simulink model "MultiLoop_mode1_old"  (R2021b)
settings: Solver=ode45  StartTime=0.0  StopTime=72  FixedStep=Ts_base  MinStep=1e-6  RelTol=1e-6
PreLoadFcn:
  | Mode_1_Init
InitFcn:
  | hApp = TEP_app;
  | %hApp = fault_selection_App;
StartFcn:
  | disp('simulator')
  | blk = 'MultiLoop_mode1/TE Plant/Pressure';
  | event = 'PostOutputs';
  | listener = @(app, event) updateGUI(hApp);
  | h = add_exec_event_listener(blk, event, listener);
StopFcn:
  | %TEplot
undefined symbols (not defined in the file or in its folder): r1_0, r4_0, Ts_base, Ts_save
libraries: TElib x17
settings Model: PacingRate=0.001000  Creator=ricker  LastModifiedBy=Omar
settings SolverCC: AlgebraicLoopSolver=TrustRegion
settings DataIOCC: LoadInitialState=on  SaveFinalState=on  SaveFormat=Structure  SignalLoggingSaveFormat=ModelDataLogs  SaveOutput=off  SignalLogging=off  SaveTime=off  ReturnWorkspaceOutputs=off  SignalLoggingName=sigsOut
settings OptimizationCC: InitFltsAndDblsToZero=on  LifeSpan=inf
settings DebuggingCC: SaveWithParameterizedLinksMsg=none  UnderspecifiedInitializationDetection=Classic  MergeDetectMultiDrivingBlocksExec=none  SignalResolutionControl=TryResolveAllWithWarning  MultiTaskDSMMsg=warning  MultiTaskCondExecSysMsg=none  FcnCallInpInsideContextMsg=warning  SFUnexpectedBacktrackingDiag=warning  SFNoUnconditionalDefaultTransitionDiag=warning  SFExecutionAtInitializationDiag=none  SFMachineParentedDataDiag=warning  ArithmeticOperatorsInVariantConditions=warning
settings HardwareCC: ProdBitPerPointer=32  ProdBitPerSizeT=32  ProdBitPerPtrDiffT=32  ProdLargestAtomicFloat=None  ProdIntDivRoundTo=Undefined  ProdEndianess=Unspecified  ProdWordSize=32  ProdHWDeviceType=32-bit Generic  TargetUnknown=on
settings ModelReferenceCC: PropagateSignalLabelsOutOfModel=off
settings SFSimCC: SimUseLocalCustomCode=off  CustomCodeUndefinedFunction=UseInterfaceOnly
settings RTWCC: RTWUseLocalCustomCode=off
settings CodeAppCC: StateflowObjectComments=on
settings GRTTargetCC: TargetFcnLib=ansi_tfl_tmw.mat  TargetLangStandard=C89/C90 (ANSI)  CombineOutputUpdateFcns=off  GRTInterface=on
settings ConfigComp: CovMetricSettings=dw  CovSaveCumulativeToWorkspaceVar=on  CovSaveSingleToWorkspaceVar=on  CovExternalEMLEnable=off  CovSFcnEnable=off

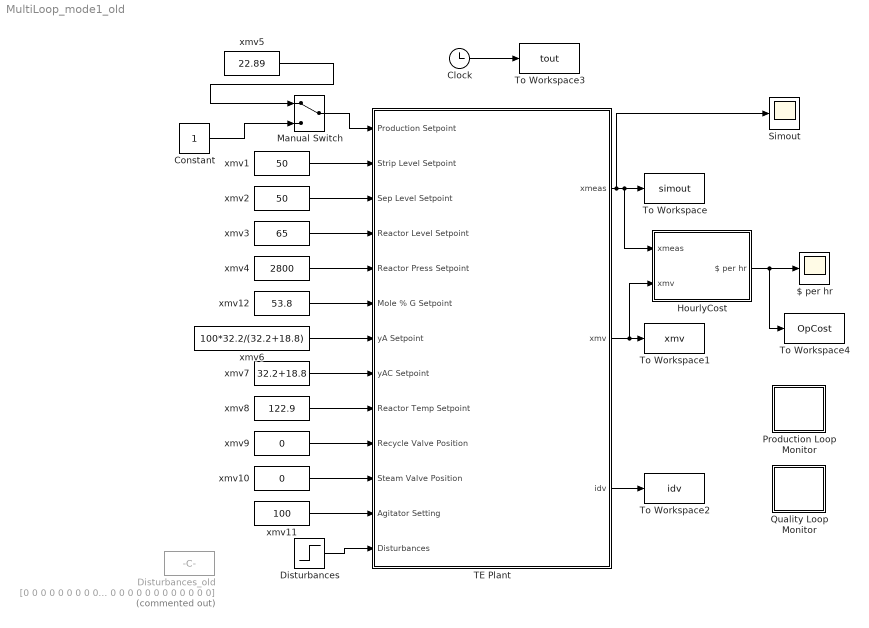
== system MultiLoop_mode1_old ==
  $ per hr : Scope
  Clock : Clock
  Constant : Constant
  Disturbances : Step  Time=0  Before=[0 0 0 0 0 0 0 0 0 0 0 0 0 0 0 0 0 0 0 0 0 0 0 0 0 0 0 0]  After=[0 0 0 0 0 0 0 0 0 0 0 0 0 0 0 0 0 0 0 0 0 0 0 0 0 0 0 0]  SampleTime=0
  Disturbances_old : Constant  Commented=on  Value=[0 0 0 0 0 0 0 0 0 0 0 0 0 0 0 0 0 0 0 0 0 0 0 0 0 0 0 0]
  HourlyCost : Subsystem
  Manual Switch : ManualSwitch
  Production Loop Monitor : Subsystem
  Quality Loop Monitor : Subsystem
  Simout : Scope
  TE Plant : Subsystem
  To Workspace : ToWorkspace  VariableName=simout  SampleTime=Ts_save
  To Workspace1 : ToWorkspace  VariableName=xmv  SampleTime=Ts_save
  To Workspace2 : ToWorkspace  VariableName=idv  SampleTime=Ts_save
  To Workspace3 : ToWorkspace  VariableName=tout  SampleTime=Ts_save
  To Workspace4 : ToWorkspace  VariableName=OpCost  SampleTime=Ts_save
  xmv1 : Constant  Value=50
  xmv10 : Constant  Value=0
  xmv11 : Constant  Value=100
  xmv12 : Constant  Value=53.8
  xmv2 : Constant  Value=50
  xmv3 : Constant  Value=65
  xmv4 : Constant  Value=2800
  xmv5 : Constant  Value=22.89
  xmv6 : Constant  Value=100*32.2/(32.2+18.8)
  xmv7 : Constant  Value=32.2+18.8
  xmv8 : Constant  Value=122.9
  xmv9 : Constant  Value=0
  wires:
  TE Plant/1(xmeas) -> Simout/1, To Workspace/1, HourlyCost/1(xmeas)
  xmv1/1 -> TE Plant/2(Strip Level Setpoint)
  xmv2/1 -> TE Plant/3(Sep Level Setpoint)
  xmv3/1 -> TE Plant/4(Reactor Level Setpoint)
  xmv4/1 -> TE Plant/5(Reactor Press Setpoint)
  xmv8/1 -> TE Plant/9(Reactor Temp Setpoint)
  xmv6/1 -> TE Plant/7(yA Setpoint)
  xmv7/1 -> TE Plant/8(yAC Setpoint)
  TE Plant/2(xmv) -> To Workspace1/1, HourlyCost/2(xmv)
  TE Plant/3(idv) -> To Workspace2/1
  Clock/1 -> To Workspace3/1
  HourlyCost/1($ per hr) -> $ per hr/1, To Workspace4/1
  xmv9/1 -> TE Plant/10(Recycle Valve Position)
  xmv10/1 -> TE Plant/11(Steam Valve Position)
  xmv11/1 -> TE Plant/12(Agitator Setting)
  xmv12/1 -> TE Plant/6(Mole % G Setpoint)
  xmv5/1 -> Manual Switch/1
  Disturbances/1 -> TE Plant/13(Disturbances)
  Constant/1 -> Manual Switch/2
  Manual Switch/1 -> TE Plant/1(Production Setpoint)

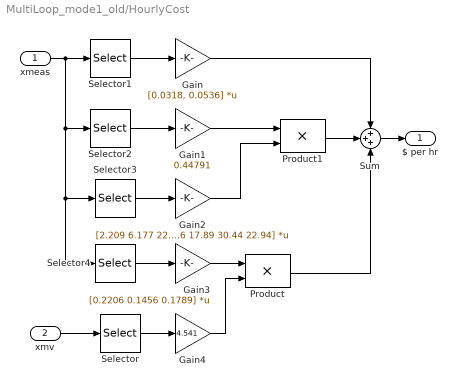
== system MultiLoop_mode1_old/HourlyCost ==
  xmeas : Inport  PortDimensions=41
  xmv : Inport  Port=2  PortDimensions=12
  Gain : Gain  Gain=[0.0318, 0.0536]  Multiplication=Matrix(K*u)  SaturateOnIntegerOverflow=on  OutDataTypeStr=Inherit: Same as input  ParamDataTypeStr=Inherit: Same as input
  Gain1 : Gain  Gain=0.44791  SaturateOnIntegerOverflow=on  OutDataTypeStr=Inherit: Same as input  ParamDataTypeStr=Inherit: Same as input
  Gain2 : Gain  Gain=[2.209 6.177 22.06 14.56 17.89 30.44 22.94]  Multiplication=Matrix(K*u)  SaturateOnIntegerOverflow=on  OutDataTypeStr=Inherit: Same as input  ParamDataTypeStr=Inherit: Same as input
  Gain3 : Gain  Gain=[0.2206 0.1456 0.1789]  Multiplication=Matrix(K*u)  SaturateOnIntegerOverflow=on  OutDataTypeStr=Inherit: Same as input  ParamDataTypeStr=Inherit: Same as input
  Gain4 : Gain  Gain=4.541  SaturateOnIntegerOverflow=on  OutDataTypeStr=Inherit: Same as input  ParamDataTypeStr=Inherit: Same as input
  Product : Product  SaturateOnIntegerOverflow=on  OutDataTypeStr=Inherit: Same as first input
  Product1 : Product  SaturateOnIntegerOverflow=on  OutDataTypeStr=Inherit: Same as first input
  Selector : Selector  InputPortWidth=12  IndexOptions=Index vector (dialog)  Indices=8  OutputSizes=1
  Selector1 : Selector  InputPortWidth=41  IndexOptions=Index vector (dialog)  Indices=[19 20]  OutputSizes=1
  Selector2 : Selector  InputPortWidth=41  IndexOptions=Index vector (dialog)  Indices=[10]  OutputSizes=1
  Selector3 : Selector  InputPortWidth=41  IndexOptions=Index vector (dialog)  Indices=[29, 31:36]  OutputSizes=1
  Selector4 : Selector  InputPortWidth=41  IndexOptions=Index vector (dialog)  Indices=[37:39]  OutputSizes=1
  Sum : Sum  Inputs=+++  SaturateOnIntegerOverflow=on
  $ per hr : Outport
  wires:
  xmv/1 -> Selector/1
  xmeas/1 -> Selector1/1, Selector2/1, Selector3/1, Selector4/1
  Selector1/1 -> Gain/1
  Selector2/1 -> Gain1/1
  Selector3/1 -> Gain2/1
  Selector4/1 -> Gain3/1
  Selector/1 -> Gain4/1
  Gain3/1 -> Product/1
  Gain4/1 -> Product/2
  Sum/1 -> $ per hr/1
  Product/1 -> Sum/3
  Gain/1 -> Sum/1
  Product1/1 -> Sum/2
  Gain1/1 -> Product1/1
  Gain2/1 -> Product1/2

== system MultiLoop_mode1_old/Production Loop Monitor ==
  Mux2 : Mux  Inputs=2
  Production : Scope
  wires:
  Mux2/1 -> Production/1
  [xmeas17] -> Mux2/2
  [Prodsp] -> Mux2/1

== system MultiLoop_mode1_old/Quality Loop Monitor ==
  Mux2 : Mux  Inputs=2
  Quality : Scope
  wires:
  [PctGsp] -> Mux2/1
  [xmeas40] -> Mux2/2
  Mux2/1 -> Quality/1

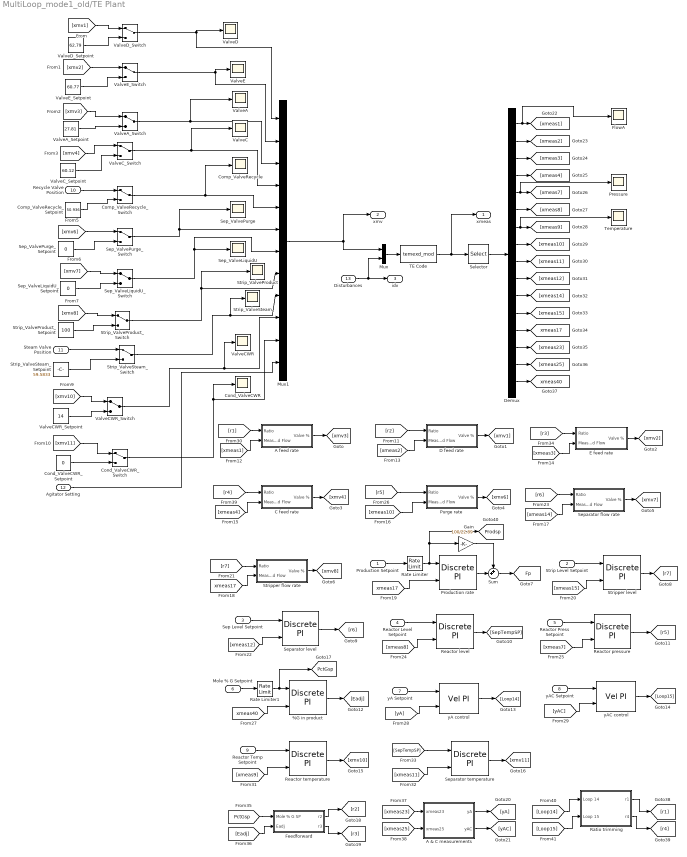
== system MultiLoop_mode1_old/TE Plant ==
  Production Setpoint : Inport
  Strip Level Setpoint : Inport  Port=2
  Sep Level Setpoint : Inport  Port=3
  Reactor Level Setpoint : Inport  Port=4
  Reactor Press Setpoint : Inport  Port=5
  Mole % G Setpoint : Inport  Port=6
  yA Setpoint : Inport  Port=7
  yAC Setpoint : Inport  Port=8
  Reactor Temp Setpoint : Inport  Port=9
  Recycle Valve Position : Inport  Port=10
  Steam Valve Position : Inport  Port=11
  Agitator Setting : Inport  Port=12
  Disturbances : Inport  Port=13
  %G in product : TElib/Discrete PI  Kc=-0.4  Ti=100/60  Ts=Ts_base  x0=Eadj_0  Hi=inf  Lo=-inf
  A & C measurements : Subsystem
  A feed rate : Subsystem
  C feed rate : Subsystem
  Comp_ValveRecycle : Scope
  Comp_ValveRecycle_Setpoint : Constant  Value=50.936
  Comp_ValveRecycle_Switch : ManualSwitch
  Cond_ValveCWR : Scope
  Cond_ValveCWR_Setpoint : Constant  Value=0
  Cond_ValveCWR_Switch : ManualSwitch
  D feed rate : Subsystem
  Demux : Demux  Outputs=16
      settings: DisplayOption=none
  E feed rate : Subsystem
  Feedforward : Subsystem
  FlowA : Scope
  Gain : Gain  Gain=100/22.89  SaturateOnIntegerOverflow=on  OutDataTypeStr=Inherit: Same as input  ParamDataTypeStr=Inherit: Same as input
  Mux : Mux  Inputs=2
  Mux1 : Mux  Inputs=12
  Pressure : Scope
  Production rate : TElib/Discrete PI  Kc=3.2  Ti=120/60  Ts=Ts_base  x0=0  Hi=30  Lo=-30
  Purge rate : Subsystem
  Rate Limiter : RateLimiter  RisingSlewLimit=0.3*22.95/24  FallingSlewLimit=-0.3*22.95/24
  Rate Limiter1 : RateLimiter  RisingSlewLimit=50/24  FallingSlewLimit=-50/24
  Ratio trimming : Subsystem
  Reactor level : TElib/Discrete PI  Kc=0.8  Ti=60/60  Ts=Ts_base  x0=SP17_0  Hi=120  Lo=0
  Reactor pressure : TElib/Discrete PI  Kc=-1e-4  Ti=20/60  Ts=Ts_base  x0=r5_0  Hi=100  Lo=0
  Reactor temperature : TElib/Discrete PI  Kc=-8  Ti=7.5/60  Ts=Ts_base  x0=xmv10_0  Hi=100  Lo=0
  Selector : Selector  InputPortWidth=41  IndexOptions=Index vector (dialog)  Indices=[1:4, 7:12, 14, 15, 17, 23, 25, 40]  OutputSizes=1
  Sep_ValveLiquidU : Scope
  Sep_ValveLiquidU_Setpoint : Constant  Value=0
  Sep_ValveLiquidU_Switch : ManualSwitch
  Sep_ValvePurge : Scope
  Sep_ValvePurge_Setpoint : Constant  Value=0
  Sep_ValvePurge_Switch : ManualSwitch
  Separator flow rate : Subsystem
  Separator level : TElib/Discrete PI  Kc=-1e-3  Ti=200/60  Ts=Ts_base  x0=r6_0  Hi=100  Lo=0
  Separator temperature : TElib/Discrete PI  Kc=-4  Ti=15/60  Ts=Ts_base  x0=xmv11_0  Hi=100  Lo=0
  Strip_ValveProduct : Scope
  Strip_ValveProduct_Setpoint : Constant  Value=100
  Strip_ValveProduct_Switch : ManualSwitch
  Strip_ValveSteam : Scope
  Strip_ValveSteam_Setpoint : Constant  Value=59.5833
  Strip_ValveSteam_Switch : ManualSwitch
  Stripper flow rate : Subsystem
  Stripper level : TElib/Discrete PI  Kc=-2e-4  Ti=200/60  Ts=Ts_base  x0=r7_0  Hi=100  Lo=0
  Sum : Sum  Inputs=++|  SaturateOnIntegerOverflow=on
  TE Code : S-Function  FunctionName=temexd_mod  SFunctionDeploymentMode=off  EnableBusSupport=off
  Temperature : Scope
  ValveA : Scope
  ValveA_Setpoint : Constant  Value=27.81
  ValveA_Switch : ManualSwitch
  ValveC : Scope
  ValveCWR : Scope
  ValveCWR_Setpoint : Constant  Value=14
  ValveCWR_Switch : ManualSwitch
  ValveC_Setpoint : Constant  Value=60.12
  ValveC_Switch : ManualSwitch
  ValveD : Scope
  ValveD_Setpoint : Constant  Value=62.79
  ValveD_Switch : ManualSwitch
  ValveE : Scope
  ValveE_Setpoint : Constant  Value=60.77
  ValveE_Switch : ManualSwitch
  yA control : TElib/Discrete PI/Vel PI  Kc=2e-4  Ti=1  Ts=0.1
  yAC control : TElib/Discrete PI/Vel PI  Kc=3e-4  Ti=2  Ts=0.1
  xmeas : Outport
  xmv : Outport  Port=2
  idv : Outport  Port=3
  tag scope: Fp=global, PctGsp=global, Prodsp=global, xmeas17=global, xmeas40=global
  wires:
  Mux/1 -> TE Code/1
  Disturbances/1 -> Mux/2, idv/1
  TE Code/1 -> xmeas/1, Selector/1
  [xmv1] -> ValveD_Switch/1
  Recycle Valve Position/1 -> Comp_ValveRecycle_Switch/1
  [xmv6] -> Sep_ValvePurge_Switch/1
  [xmv7] -> Sep_ValveLiquidU_Switch/1
  [xmv8] -> Strip_ValveProduct_Switch/1
  Steam Valve Position/1 -> Strip_ValveSteam_Switch/1
  [xmv10] -> ValveCWR_Switch/1
  [xmv11] -> Cond_ValveCWR_Switch/1
  Agitator Setting/1 -> Mux1/12
  A feed rate/1(Valve %) -> [xmv3]
  [xmeas1] -> A feed rate/2(Measured Flow)
  D feed rate/1(Valve %) -> [xmv1]
  [xmeas2] -> D feed rate/2(Measured Flow)
  E feed rate/1(Valve %) -> [xmv2]
  [xmeas3] -> E feed rate/2(Measured Flow)
  C feed rate/1(Valve %) -> [xmv4]
  [xmeas4] -> C feed rate/2(Measured Flow)
  Purge rate/1(Valve %) -> [xmv6]
  [xmeas10] -> Purge rate/2(Measured Flow)
  Separator flow rate/1(Valve %) -> [xmv7]
  [xmeas14] -> Separator flow rate/2(Measured Flow)
  Stripper flow rate/1(Valve %) -> [xmv8]
  [xmeas17] -> Stripper flow rate/2(Measured Flow)
  [xmeas17] -> Production rate/2
  [xmeas15] -> Stripper level/2
  Strip Level Setpoint/1 -> Stripper level/1
  Stripper level/1 -> [r7]
  [r7] -> Stripper flow rate/1(Ratio)
  [xmeas12] -> Separator level/2
  Sep Level Setpoint/1 -> Separator level/1
  Separator level/1 -> [r6]
  [r6] -> Separator flow rate/1(Ratio)
  [xmeas8] -> Reactor level/2
  Reactor Level Setpoint/1 -> Reactor level/1
  Reactor level/1 -> [SepTempSP]
  [xmeas7] -> Reactor pressure/2
  Reactor Press Setpoint/1 -> Reactor pressure/1
  Reactor pressure/1 -> [r5]
  [r5] -> Purge rate/1(Ratio)
  [xmeas40] -> %G in product/2
  %G in product/1 -> [Eadj]
  [yA] -> yA control/2
  yA Setpoint/1 -> yA control/1
  yA control/1 -> [Loop14]
  [yAC] -> yAC control/2
  yAC Setpoint/1 -> yAC control/1
  yAC control/1 -> [Loop15]
  [r1] -> A feed rate/1(Ratio)
  [xmeas9] -> Reactor temperature/2
  Reactor Temp Setpoint/1 -> Reactor temperature/1
  Reactor temperature/1 -> [xmv10]
  [xmeas11] -> Separator temperature/2
  [SepTempSP] -> Separator temperature/1
  Separator temperature/1 -> [xmv11]
  [r3] -> E feed rate/1(Ratio)
  [PctGsp] -> Feedforward/1(Mole % G SP)
  [Eadj] -> Feedforward/2(Eadj)
  Feedforward/1(r2) -> [r2]
  Feedforward/2(r3) -> [r3]
  [xmeas23] -> A & C measurements/1(xmeas23)
  [xmeas25] -> A & C measurements/2(xmeas25)
  A & C measurements/1(yA) -> [yA]
  A & C measurements/2(yAC) -> [yAC]
  Mux1/1 -> Mux/1, xmv/1
  Selector/1 -> Demux/1
  Demux/1 -> FlowA/1, [xmeas1]
  Demux/2 -> [xmeas2]
  Demux/3 -> [xmeas3]
  Demux/4 -> [xmeas4]
  Demux/5 -> [xmeas7], Pressure/1
  Demux/6 -> [xmeas8]
  Demux/7 -> [xmeas9], Temperature/1
  Demux/8 -> [xmeas10]
  Demux/9 -> [xmeas11]
  Demux/10 -> [xmeas12]
  Demux/11 -> [xmeas14]
  Demux/12 -> [xmeas15]
  Demux/13 -> [xmeas17]
  Demux/14 -> [xmeas23]
  Demux/15 -> [xmeas25]
  Demux/16 -> [xmeas40]
  [r4] -> C feed rate/1(Ratio)
  [Loop14] -> Ratio trimming/1(Loop 14)
  [Loop15] -> Ratio trimming/2(Loop 15)
  Ratio trimming/1(r1) -> [r1]
  Ratio trimming/2(r4) -> [r4]
  Production Setpoint/1 -> Rate Limiter/1
  Rate Limiter/1 -> Production rate/1, [Prodsp], Gain/1
  Mole % G Setpoint/1 -> Rate Limiter1/1
  Rate Limiter1/1 -> %G in product/1, [PctGsp]
  Production rate/1 -> Sum/2
  Sum/1 -> [Fp]
  Gain/1 -> Sum/1
  ValveD_Setpoint/1 -> ValveD_Switch/2
  ValveD_Switch/1 -> Mux1/1, ValveD/1
  Cond_ValveCWR_Setpoint/1 -> Cond_ValveCWR_Switch/2
  Cond_ValveCWR_Switch/1 -> Cond_ValveCWR/1, Mux1/11
  Sep_ValvePurge_Setpoint/1 -> Sep_ValvePurge_Switch/2
  Sep_ValvePurge_Switch/1 -> Mux1/6, Sep_ValvePurge/1
  Sep_ValveLiquidU_Setpoint/1 -> Sep_ValveLiquidU_Switch/2
  Sep_ValveLiquidU_Switch/1 -> Mux1/7, Sep_ValveLiquidU/1
  Comp_ValveRecycle_Switch/1 -> Comp_ValveRecycle/1, Mux1/5
  Comp_ValveRecycle_Setpoint/1 -> Comp_ValveRecycle_Switch/2
  [xmv3] -> ValveA_Switch/1
  ValveA_Switch/1 -> Mux1/3, ValveA/1
  ValveA_Setpoint/1 -> ValveA_Switch/2
  ValveE_Switch/1 -> Mux1/2, ValveE/1
  [xmv2] -> ValveE_Switch/1
  [xmv4] -> ValveC_Switch/1
  ValveC_Switch/1 -> ValveC/1, Mux1/4
  ValveC_Setpoint/1 -> ValveC_Switch/2
  Strip_ValveProduct_Setpoint/1 -> Strip_ValveProduct_Switch/2
  Strip_ValveProduct_Switch/1 -> Strip_ValveProduct/1, Mux1/8
  ValveCWR_Setpoint/1 -> ValveCWR_Switch/2
  ValveCWR_Switch/1 -> ValveCWR/1, Mux1/10
  Strip_ValveSteam_Switch/1 -> Strip_ValveSteam/1, Mux1/9
  Strip_ValveSteam_Setpoint/1 -> Strip_ValveSteam_Switch/2
  ValveE_Setpoint/1 -> ValveE_Switch/2
  [r2] -> D feed rate/1(Ratio)

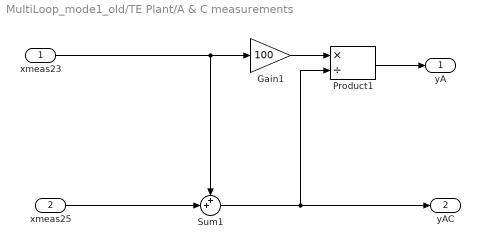
== system MultiLoop_mode1_old/TE Plant/A & C measurements ==
  xmeas23 : Inport
  xmeas25 : Inport  Port=2
  Gain1 : Gain  Gain=100  SaturateOnIntegerOverflow=on  OutDataTypeStr=Inherit: Same as input  ParamDataTypeStr=Inherit: Same as input
  Product1 : Product  Inputs=*/  SaturateOnIntegerOverflow=on  OutDataTypeStr=Inherit: Same as first input
  Sum1 : Sum  Inputs=++|  SaturateOnIntegerOverflow=on
  yA : Outport
  yAC : Outport  Port=2
  wires:
  Sum1/1 -> yAC/1, Product1/2
  xmeas23/1 -> Sum1/1, Gain1/1
  xmeas25/1 -> Sum1/2
  Gain1/1 -> Product1/1
  Product1/1 -> yA/1

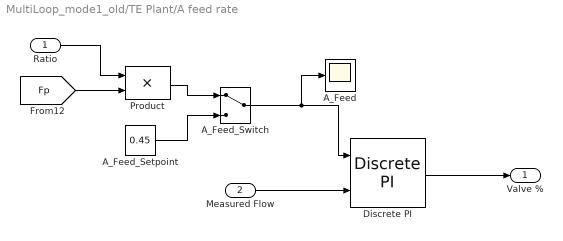
== system MultiLoop_mode1_old/TE Plant/A feed rate ==
  Ratio : Inport
  Measured Flow : Inport  Port=2
  A_Feed : Scope
  A_Feed_Setpoint : Constant  Value=0.45
  A_Feed_Switch : ManualSwitch
  Discrete PI : TElib/Discrete PI  Kc=0.01  Ti=0.001/60  Ts=Ts_base  x0=xmv3_0  Hi=100  Lo=0
  Product : Product  SaturateOnIntegerOverflow=on  OutDataTypeStr=Inherit: Same as first input
  Valve % : Outport
  wires:
  Discrete PI/1 -> Valve %/1
  Ratio/1 -> Product/1
  [Fp] -> Product/2
  Measured Flow/1 -> Discrete PI/2
  Product/1 -> A_Feed_Switch/1
  A_Feed_Setpoint/1 -> A_Feed_Switch/2
  A_Feed_Switch/1 -> Discrete PI/1, A_Feed/1

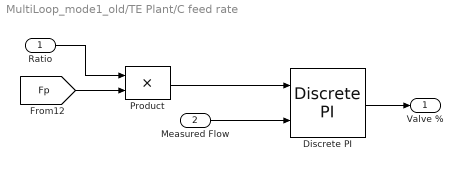
== system MultiLoop_mode1_old/TE Plant/C feed rate ==
  Ratio : Inport
  Measured Flow : Inport  Port=2
  Discrete PI : TElib/Discrete PI  Kc=0.003  Ti=0.001/60  Ts=Ts_base  x0=xmv4_0  Hi=100  Lo=0
  Product : Product  SaturateOnIntegerOverflow=on  OutDataTypeStr=Inherit: Same as first input
  Valve % : Outport
  wires:
  Product/1 -> Discrete PI/1
  Measured Flow/1 -> Discrete PI/2
  [Fp] -> Product/2
  Ratio/1 -> Product/1
  Discrete PI/1 -> Valve %/1

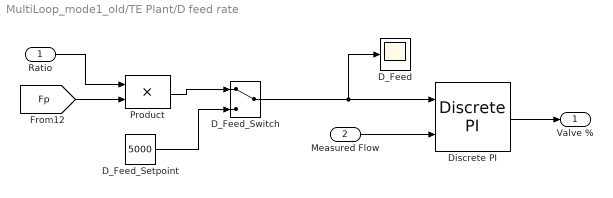
== system MultiLoop_mode1_old/TE Plant/D feed rate ==
  Ratio : Inport
  Measured Flow : Inport  Port=2
  D_Feed : Scope
  D_Feed_Setpoint : Constant  Value=5000
  D_Feed_Switch : ManualSwitch
  Discrete PI : TElib/Discrete PI  Kc=1.6e-6  Ti=0.001/60  Ts=Ts_base  x0=xmv1_0  Hi=100  Lo=0
  Product : Product  SaturateOnIntegerOverflow=on  OutDataTypeStr=Inherit: Same as first input
  Valve % : Outport
  wires:
  Product/1 -> D_Feed_Switch/1
  Measured Flow/1 -> Discrete PI/2
  [Fp] -> Product/2
  Ratio/1 -> Product/1
  Discrete PI/1 -> Valve %/1
  D_Feed_Setpoint/1 -> D_Feed_Switch/2
  D_Feed_Switch/1 -> D_Feed/1, Discrete PI/1

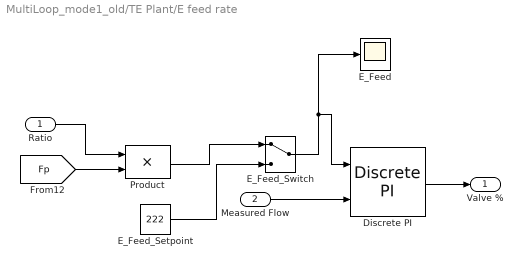
== system MultiLoop_mode1_old/TE Plant/E feed rate ==
  Ratio : Inport
  Measured Flow : Inport  Port=2
  Discrete PI : TElib/Discrete PI  Kc=1.8e-6  Ti=0.001/60  Ts=Ts_base  x0=xmv2_0  Hi=100  Lo=0
  E_Feed : Scope
  E_Feed_Setpoint : Constant  Value=222
  E_Feed_Switch : ManualSwitch
  Product : Product  SaturateOnIntegerOverflow=on  OutDataTypeStr=Inherit: Same as first input
  Valve % : Outport
  wires:
  Product/1 -> E_Feed_Switch/1
  Measured Flow/1 -> Discrete PI/2
  [Fp] -> Product/2
  Ratio/1 -> Product/1
  Discrete PI/1 -> Valve %/1
  E_Feed_Switch/1 -> E_Feed/1, Discrete PI/1
  E_Feed_Setpoint/1 -> E_Feed_Switch/2

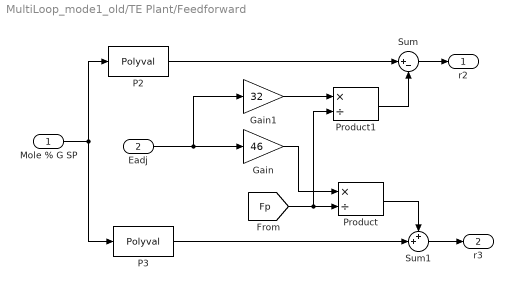
== system MultiLoop_mode1_old/TE Plant/Feedforward ==
  Mole % G SP : Inport
  Eadj : Inport  Port=2
  Gain : Gain  Gain=46  SaturateOnIntegerOverflow=on  OutDataTypeStr=Inherit: Same as input  ParamDataTypeStr=Inherit: Same as input
  Gain1 : Gain  Gain=32  SaturateOnIntegerOverflow=on  OutDataTypeStr=Inherit: Same as input  ParamDataTypeStr=Inherit: Same as input
  P2 : Polyval  Coefs="[1.5192e-003  5.9446e-001  2.7690e-001]"
  P3 : Polyval  Coefs="[-1.1377e-003 -8.0893e-001  9.1060e+001]"
  Product : Product  Inputs=*/  SaturateOnIntegerOverflow=on  OutDataTypeStr=Inherit: Same as first input
  Product1 : Product  Inputs=*/  SaturateOnIntegerOverflow=on  OutDataTypeStr=Inherit: Same as first input
  Sum : Sum  Inputs=|+-  SaturateOnIntegerOverflow=on
  Sum1 : Sum  Inputs=++|  SaturateOnIntegerOverflow=on
  r2 : Outport
  r3 : Outport  Port=2
  wires:
  Mole % G SP/1 -> P2/1, P3/1
  Sum/1 -> r2/1
  P2/1 -> Sum/1
  Sum1/1 -> r3/1
  P3/1 -> Sum1/2
  Product/1 -> Sum1/1
  [Fp] -> Product/2, Product1/2
  Gain/1 -> Product/1
  Eadj/1 -> Gain/1, Gain1/1
  Product1/1 -> Sum/2
  Gain1/1 -> Product1/1

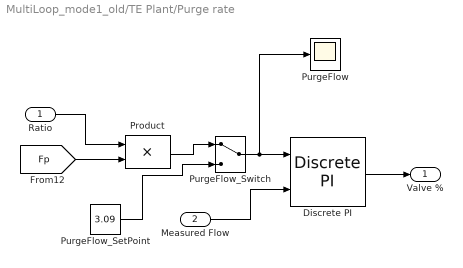
== system MultiLoop_mode1_old/TE Plant/Purge rate ==
  Ratio : Inport
  Measured Flow : Inport  Port=2
  Discrete PI : TElib/Discrete PI  Kc=0.01  Ti=0.001/60  Ts=Ts_base  x0=xmv6_0  Hi=100  Lo=0
  Product : Product  SaturateOnIntegerOverflow=on  OutDataTypeStr=Inherit: Same as first input
  PurgeFlow : Scope
  PurgeFlow_SetPoint : Constant  Value=3.09
  PurgeFlow_Switch : ManualSwitch
  Valve % : Outport
  wires:
  Discrete PI/1 -> Valve %/1
  Ratio/1 -> Product/1
  [Fp] -> Product/2
  Measured Flow/1 -> Discrete PI/2
  Product/1 -> PurgeFlow_Switch/1
  PurgeFlow_SetPoint/1 -> PurgeFlow_Switch/2
  PurgeFlow_Switch/1 -> PurgeFlow/1, Discrete PI/1

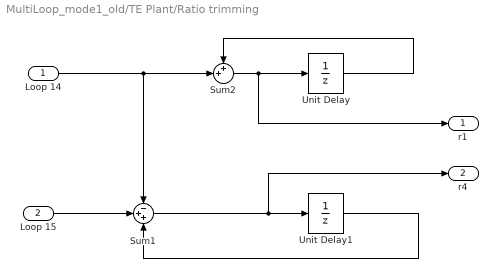
== system MultiLoop_mode1_old/TE Plant/Ratio trimming ==
  Loop 14 : Inport
  Loop 15 : Inport  Port=2
  Sum1 : Sum  Inputs=-++  SaturateOnIntegerOverflow=on
  Sum2 : Sum  Inputs=++|  SaturateOnIntegerOverflow=on
  Unit Delay : UnitDelay  InitialCondition=r1_0  SampleTime=0.1  HasFrameUpgradeWarning=on
  Unit Delay1 : UnitDelay  InitialCondition=r4_0  SampleTime=0.1  HasFrameUpgradeWarning=on
  r1 : Outport
  r4 : Outport  Port=2
  wires:
  Loop 15/1 -> Sum1/2
  Unit Delay/1 -> Sum2/1
  Unit Delay1/1 -> Sum1/3
  Sum2/1 -> Unit Delay/1, r1/1
  Loop 14/1 -> Sum2/2, Sum1/1
  Sum1/1 -> Unit Delay1/1, r4/1

== system MultiLoop_mode1_old/TE Plant/Separator flow rate ==
  Ratio : Inport
  Measured Flow : Inport  Port=2
  Discrete PI : TElib/Discrete PI  Kc=4e-4  Ti=0.001/60  Ts=Ts_base  x0=xmv7_0  Hi=100  Lo=0
  Product : Product  SaturateOnIntegerOverflow=on  OutDataTypeStr=Inherit: Same as first input
  Valve % : Outport
  wires:
  Product/1 -> Discrete PI/1
  Measured Flow/1 -> Discrete PI/2
  [Fp] -> Product/2
  Ratio/1 -> Product/1
  Discrete PI/1 -> Valve %/1

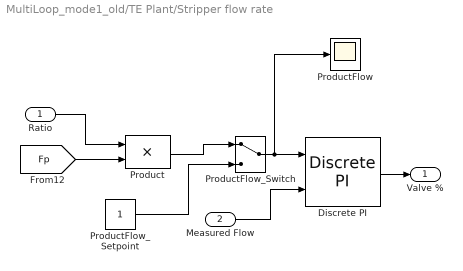
== system MultiLoop_mode1_old/TE Plant/Stripper flow rate ==
  Ratio : Inport
  Measured Flow : Inport  Port=2
  Discrete PI : TElib/Discrete PI  Kc=4e-4  Ti=0.001/60  Ts=Ts_base  x0=xmv8_0  Hi=100  Lo=0
  Product : Product  SaturateOnIntegerOverflow=on  OutDataTypeStr=Inherit: Same as first input
  ProductFlow : Scope
  ProductFlow_Setpoint : Constant
  ProductFlow_Switch : ManualSwitch
  Valve % : Outport
  wires:
  Discrete PI/1 -> Valve %/1
  Ratio/1 -> Product/1
  [Fp] -> Product/2
  Measured Flow/1 -> Discrete PI/2
  Product/1 -> ProductFlow_Switch/1
  ProductFlow_Setpoint/1 -> ProductFlow_Switch/2
  ProductFlow_Switch/1 -> ProductFlow/1, Discrete PI/1
